simulink model "ziegler_nichols_model"  (R2018b)
settings: Solver=VariableStepAuto  StartTime=0.0  StopTime=tFinal  MaxStep=.05  RelTol=1e-3
values from neighbouring files (symbols this model uses):
  G_den = [1 6 11 6]    [lecture_ziegler_nichols.m]
  G_num = [1]    [lecture_ziegler_nichols.m]
undefined symbols (not defined in the file or in its folder): KD, KI, KP
settings Model: Creator=Christopher  LastModifiedBy=Christopher

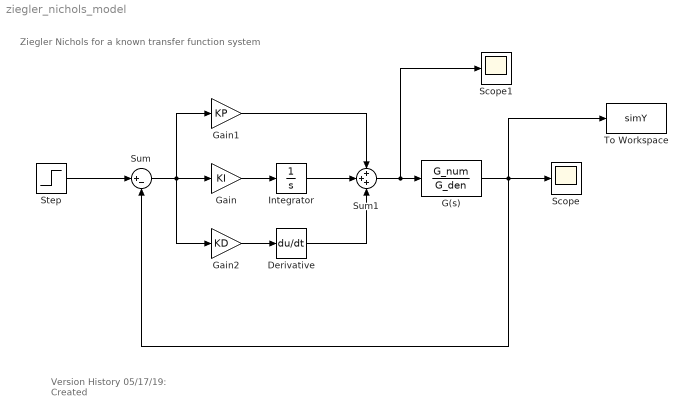
== system ziegler_nichols_model ==
  note: Version History
      | 05/17/19: Created
  note: Ziegler Nichols for a known transfer function system
  Derivative : Derivative
  G(s) : TransferFcn  Numerator=G_num  Denominator=G_den
  Gain : Gain  Gain=KI
  Gain1 : Gain  Gain=KP
  Gain2 : Gain  Gain=KD
  Integrator : Integrator
  Scope : Scope
  Scope1 : Scope
  Step : Step  SampleTime=0
  Sum : Sum  Inputs=|+-
  Sum1 : Sum  Inputs=+++
  To Workspace : ToWorkspace  VariableName=simY  SaveFormat=Timeseries  SampleTime=-1
  wires:
  Gain/1 -> Integrator/1
  G(s)/1 -> To Workspace/1, Sum/2, Scope/1
  Sum/1 -> Gain2/1, Gain1/1, Gain/1
  Step/1 -> Sum/1
  Sum1/1 -> Scope1/1, G(s)/1
  Gain2/1 -> Derivative/1
  Integrator/1 -> Sum1/2
  Gain1/1 -> Sum1/1
  Derivative/1 -> Sum1/3
